simulink model "test"  (R2020a)
settings: Solver=VariableStepAuto  StartTime=0.0  StopTime=10.0  RelTol=1e-3
settings Model: Creator=seanchai  LastModifiedBy=seanchai

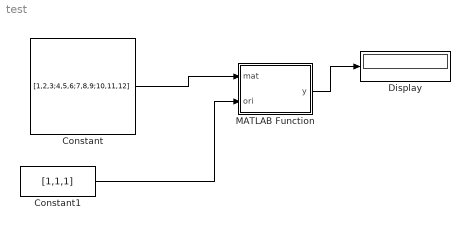
== system test ==
  Constant : Constant  Value=[1,2,3;4,5,6;7,8,9;10,11,12]
  Constant1 : Constant  Value=[1,1,1]
  Display : Display
  MATLAB Function : MATLAB Function  TreatAsAtomicUnit=on
  wires:
  Constant/1 -> MATLAB Function/1(mat)
  Constant1/1 -> MATLAB Function/2(ori)
  MATLAB Function/1(y) -> Display/1

== matlab function test/MATLAB Function ==
  data: mat input; y output; ori input
function y = fcn(mat,ori)
    rows = size(mat,2);
    u = mat - repmat(ori,rows,1);
    
y = u;
